simulink model "three_phase_diode_rectifier_with_input_filter"  (R2016a)
settings: Solver=VariableStepAuto  StartTime=0.0  StopTime=0.5  RelTol=1e-3
libraries: powerlib x54
settings Model: Creator=Gorkem  LastModifiedBy=Gorkem

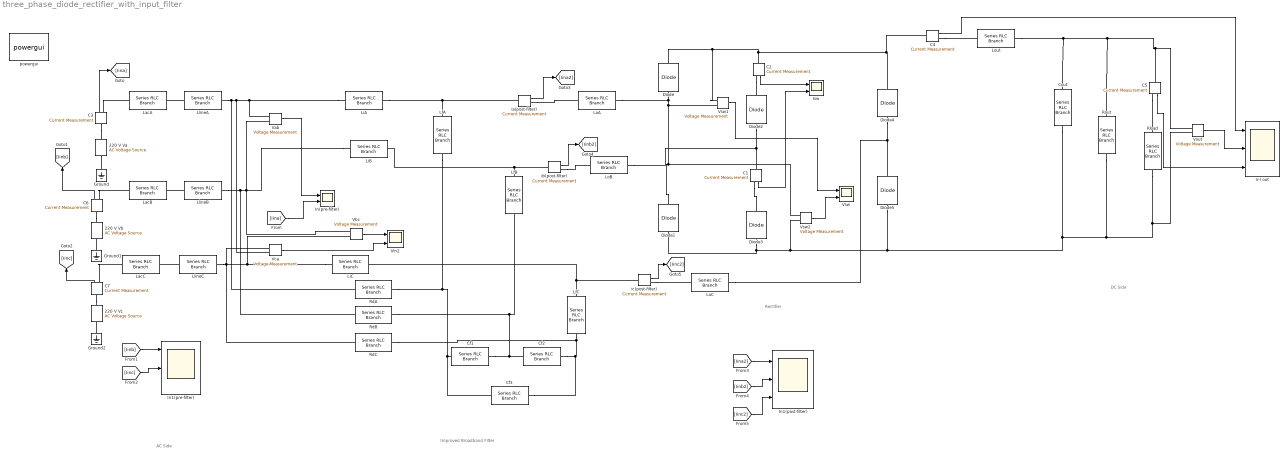
== system three_phase_diode_rectifier_with_input_filter ==
  note: Improved Broadband Filter
  note: DC Side
  note: Rectifier
  note: AC Side
  220 V Va : powerlib/Electrical Sources/AC Voltage Source  Amplitude=311  Phase=0  Frequency=50  SampleTime=0  Measurements=Voltage  BusType=swing  Pref=10e3  Qref=0  Qmin=-inf  Qmax=+inf
  220 V Vb : powerlib/Electrical Sources/AC Voltage Source  Amplitude=311  Phase=120  Frequency=50  SampleTime=0  Measurements=Voltage  BusType=swing  Pref=10e3  Qref=0  Qmin=-inf  Qmax=+inf
  220 V Vc : powerlib/Electrical Sources/AC Voltage Source  Amplitude=311  Phase=240  Frequency=50  SampleTime=0  Measurements=Voltage  BusType=swing  Pref=10e3  Qref=0  Qmin=-inf  Qmax=+inf
  C{1..7} (7 alike) : powerlib/Measurements/Current Measurement  PhasorSimulation=off  OutputType=Complex  PSBequivalent=0
  Cf1 : powerlib/Elements/Series RLC Branch  LConnTagsString=__new0  RConnTagsString=__new0  BranchType=C  Resistance=0.1  Inductance=1.7e-3  SetiL0=off  InitialCurrent=0  Capacitance=60e-6  Setx0=off  InitialVoltage=0  Measurements=Branch voltage and current
  Cf2 : powerlib/Elements/Series RLC Branch  LConnTagsString=__new0  RConnTagsString=__new0  BranchType=C  Resistance=0.1  Inductance=1.7e-3  SetiL0=off  InitialCurrent=0  Capacitance=60e-6  Setx0=off  InitialVoltage=0  Measurements=Branch voltage and current
  Cf3 : powerlib/Elements/Series RLC Branch  LConnTagsString=__new0  RConnTagsString=__new0  BranchType=C  Resistance=0.1  Inductance=1.7e-3  SetiL0=off  InitialCurrent=0  Capacitance=60e-6  Setx0=off  InitialVoltage=0  Measurements=Branch voltage and current
  Cout : powerlib/Elements/Series RLC Branch  LConnTagsString=__new0  RConnTagsString=__new0  BranchType=RC  Resistance=0.3  Inductance=1.6e-3  SetiL0=off  InitialCurrent=0  Capacitance=6e-3  Setx0=off  InitialVoltage=0  Measurements=Branch voltage and current
  Diode{,1..5} (6 alike) : powerlib/Power Electronics/Diode  Ron=0.01  Lon=0  Vf=0.7  IC=0  UseSnubber=off  Rs=5  Cs=0.1e-3  Measurements=off
  Ground : powerlib/Elements/Ground  LConnTagsString=a
  Ground1 : powerlib/Elements/Ground  LConnTagsString=a
  Ground2 : powerlib/Elements/Ground  LConnTagsString=a
  In(pre-filter) : Scope  NumInputPorts=2
  In1(post-filter) : Scope  NumInputPorts=3
  In1(pre-filter) : Scope  NumInputPorts=3
  Isw : Scope  NumInputPorts=2
  LacA : powerlib/Elements/Series RLC Branch  LConnTagsString=__new0  RConnTagsString=__new0  BranchType=RL  Resistance=0.1  Inductance=10e-3  SetiL0=off  InitialCurrent=0  Capacitance=1e-6  Setx0=off  InitialVoltage=0  Measurements=Branch voltage and current
  LacB : powerlib/Elements/Series RLC Branch  LConnTagsString=__new0  RConnTagsString=__new0  BranchType=RL  Resistance=0.1  Inductance=10e-3  SetiL0=off  InitialCurrent=0  Capacitance=1e-6  Setx0=off  InitialVoltage=0  Measurements=Branch voltage and current
  LacC : powerlib/Elements/Series RLC Branch  LConnTagsString=__new0  RConnTagsString=__new0  BranchType=RL  Resistance=0.1  Inductance=10e-3  SetiL0=off  InitialCurrent=0  Capacitance=1e-6  Setx0=off  InitialVoltage=0  Measurements=Branch voltage and current
  LfA : powerlib/Elements/Series RLC Branch  LConnTagsString=__new0  RConnTagsString=__new0  BranchType=L  Resistance=0.1  Inductance=1.7e-3  SetiL0=off  InitialCurrent=0  Capacitance=1e-6  Setx0=off  InitialVoltage=0  Measurements=Branch voltage and current
  LfB : powerlib/Elements/Series RLC Branch  LConnTagsString=__new0  RConnTagsString=__new0  BranchType=L  Resistance=0.1  Inductance=1.7e-3  SetiL0=off  InitialCurrent=0  Capacitance=1e-6  Setx0=off  InitialVoltage=0  Measurements=Branch voltage and current
  LfC : powerlib/Elements/Series RLC Branch  LConnTagsString=__new0  RConnTagsString=__new0  BranchType=L  Resistance=0.1  Inductance=1.7e-3  SetiL0=off  InitialCurrent=0  Capacitance=1e-6  Setx0=off  InitialVoltage=0  Measurements=Branch voltage and current
  LiA : powerlib/Elements/Series RLC Branch  LConnTagsString=__new0  RConnTagsString=__new0  BranchType=L  Resistance=0.1  Inductance=3.8e-3  SetiL0=off  InitialCurrent=0  Capacitance=1e-6  Setx0=off  InitialVoltage=0  Measurements=Branch voltage and current
  LiB : powerlib/Elements/Series RLC Branch  LConnTagsString=__new0  RConnTagsString=__new0  BranchType=L  Resistance=0.1  Inductance=3.8e-3  SetiL0=off  InitialCurrent=0  Capacitance=1e-6  Setx0=off  InitialVoltage=0  Measurements=Branch voltage and current
  LiC : powerlib/Elements/Series RLC Branch  LConnTagsString=__new0  RConnTagsString=__new0  BranchType=L  Resistance=0.1  Inductance=3.8e-3  SetiL0=off  InitialCurrent=0  Capacitance=1e-6  Setx0=off  InitialVoltage=0  Measurements=Branch voltage and current
  LlineA : powerlib/Elements/Series RLC Branch  LConnTagsString=__new0  RConnTagsString=__new0  BranchType=RL  Resistance=0.015  Inductance=5e-6  SetiL0=off  InitialCurrent=0  Capacitance=1e-6  Setx0=off  InitialVoltage=0  Measurements=Branch voltage and current
  LlineB : powerlib/Elements/Series RLC Branch  LConnTagsString=__new0  RConnTagsString=__new0  BranchType=RL  Resistance=0.015  Inductance=5e-6  SetiL0=off  InitialCurrent=0  Capacitance=1e-6  Setx0=off  InitialVoltage=0  Measurements=Branch voltage and current
  LlineC : powerlib/Elements/Series RLC Branch  LConnTagsString=__new0  RConnTagsString=__new0  BranchType=RL  Resistance=0.015  Inductance=5e-6  SetiL0=off  InitialCurrent=0  Capacitance=1e-6  Setx0=off  InitialVoltage=0  Measurements=Branch voltage and current
  LoA : powerlib/Elements/Series RLC Branch  LConnTagsString=__new0  RConnTagsString=__new0  BranchType=L  Resistance=0.1  Inductance=1.1e-3  SetiL0=off  InitialCurrent=0  Capacitance=1e-6  Setx0=off  InitialVoltage=0  Measurements=Branch voltage and current
  LoB : powerlib/Elements/Series RLC Branch  LConnTagsString=__new0  RConnTagsString=__new0  BranchType=L  Resistance=0.1  Inductance=1.1e-3  SetiL0=off  InitialCurrent=0  Capacitance=1e-6  Setx0=off  InitialVoltage=0  Measurements=Branch voltage and current
  LoC : powerlib/Elements/Series RLC Branch  LConnTagsString=__new0  RConnTagsString=__new0  BranchType=L  Resistance=0.1  Inductance=1.1e-3  SetiL0=off  InitialCurrent=0  Capacitance=1e-6  Setx0=off  InitialVoltage=0  Measurements=Branch voltage and current
  "Lout " : powerlib/Elements/Series RLC Branch  LConnTagsString=__new0  RConnTagsString=__new0  BranchType=RL  Resistance=0.2e-3  Inductance=20e-3  SetiL0=off  InitialCurrent=0  Capacitance=1e-6  Setx0=off  InitialVoltage=0  Measurements=Branch voltage and current
  RdA : powerlib/Elements/Series RLC Branch  LConnTagsString=__new0  RConnTagsString=__new0  BranchType=R  Resistance=10  Inductance=10e-3  SetiL0=off  InitialCurrent=0  Capacitance=1e-6  Setx0=off  InitialVoltage=0  Measurements=Branch voltage and current
  RdB : powerlib/Elements/Series RLC Branch  LConnTagsString=__new0  RConnTagsString=__new0  BranchType=R  Resistance=10  Inductance=10e-3  SetiL0=off  InitialCurrent=0  Capacitance=1e-6  Setx0=off  InitialVoltage=0  Measurements=Branch voltage and current
  RdC : powerlib/Elements/Series RLC Branch  LConnTagsString=__new0  RConnTagsString=__new0  BranchType=R  Resistance=10  Inductance=10e-3  SetiL0=off  InitialCurrent=0  Capacitance=1e-6  Setx0=off  InitialVoltage=0  Measurements=Branch voltage and current
  Rload : powerlib/Elements/Series RLC Branch  LConnTagsString=__new0  RConnTagsString=__new0  BranchType=R  Resistance=150  Inductance=1.6e-3  SetiL0=off  InitialCurrent=0  Capacitance=1e-6  Setx0=off  InitialVoltage=0  Measurements=Branch voltage and current
  Rout : powerlib/Elements/Series RLC Branch  LConnTagsString=__new0  RConnTagsString=__new0  BranchType=R  Resistance=10  Inductance=1.6e-3  SetiL0=off  InitialCurrent=0  Capacitance=1e-6  Setx0=off  InitialVoltage=0  Measurements=Branch voltage and current
  V-I out : Scope  NumInputPorts=3
  Vab : powerlib/Measurements/Voltage Measurement  PhasorSimulation=off  OutputType=Complex  PSBequivalent=0
  Vbc : powerlib/Measurements/Voltage Measurement  PhasorSimulation=off  OutputType=Complex  PSBequivalent=0
  Vca : powerlib/Measurements/Voltage Measurement  PhasorSimulation=off  OutputType=Complex  PSBequivalent=0
  Vin2 : Scope  NumInputPorts=2
  Vout : powerlib/Measurements/Voltage Measurement  PhasorSimulation=off  OutputType=Complex  PSBequivalent=0
  Vsw : Scope  NumInputPorts=2
  Vsw1 : powerlib/Measurements/Voltage Measurement  PhasorSimulation=off  OutputType=Complex  PSBequivalent=0
  Vsw2 : powerlib/Measurements/Voltage Measurement  PhasorSimulation=off  OutputType=Complex  PSBequivalent=0
  ia(post-filter) : powerlib/Measurements/Current Measurement  PhasorSimulation=off  OutputType=Complex  PSBequivalent=0
  ib(post-filter) : powerlib/Measurements/Current Measurement  PhasorSimulation=off  OutputType=Complex  PSBequivalent=0
  ic(post-filter) : powerlib/Measurements/Current Measurement  PhasorSimulation=off  OutputType=Complex  PSBequivalent=0
  powergui : powerlib/powergui  Priority=1  SimulationMode=Continuous  SolverType=Tustin/Backward Euler (TBE)  SampleTime=50e-6  frequency=60  SPID=off  DisableSnubberDevices=on  DisableRonSwitches=off  DisableVfSwitches=off  SwTol=0  DisplayEquations=off  Interpol=off  ExternalGateDelay=off  methode=off  Ts=10  FunctionMessages=on  echomessages=on  HookPort=off  EnableUseOfTLC=off  x0status=blocks  frequencyindice=0  Pbase=250  ErrMax=1e-4  Iterations=50  UnitsV=V  UnitsW=W  buscounter=0  RestoreLinks=warning  ResistiveCurrentMeasurement=off  Frange=[0:2:500]  Ylog=off  Xlog=on  ShowGrid=off  save=off  variable=ZData  structure=0  ZoomFFT=off  StartTime=0.0  cycles=1  DisplayStyle=1  fundamental=60  FreqAxis=off  MaxFrequency=1000  frequencyindicesteady=1  RmsSteady=1  display=off
  wires:
  Vab/1 -> In(pre-filter)/1
  C2/1 -> Isw/1
  C1/1 -> Isw/2
  C3/1 -> [Iina]
  [Iina] -> In(pre-filter)/2
  Vout/1 -> V-I out/2
  C4/1 -> V-I out/1
  Vsw1/1 -> Vsw/1
  Vsw2/1 -> Vsw/2
  C5/1 -> V-I out/3
  [Iinb] -> In1(pre-filter)/1
  [Iinc] -> In1(pre-filter)/2
  C6/1 -> [Iinb]
  C7/1 -> [Iinc]
  Vbc/1 -> Vin2/1
  Vca/1 -> Vin2/2
  ia(post-filter)/1 -> [Iina2]
  ib(post-filter)/1 -> [Iinb2]
  ic(post-filter)/1 -> [Iinc2]
  [Iina2] -> In1(post-filter)/1
  [Iinb2] -> In1(post-filter)/2
  [Iinc2] -> In1(post-filter)/3
  connections:
  LlineA/LConn1 -- LacA/RConn1
  Diode4/RConn1 -- C4/LConn1 -- Diode/RConn1 -- Vsw1/LConn1 -- C2/LConn1
  Diode3/LConn1 -- Rout/RConn1 -- Vout/LConn2 -- Rload/RConn1 -- Cout/RConn1 -- Diode5/LConn1 -- Vsw2/LConn2 -- Diode1/LConn1
  LiA/LConn1 -- LlineA/RConn1 -- RdA/LConn1 -- Vca/LConn2 -- Vab/LConn1
  C2/RConn1 -- Diode2/RConn1
  C3/LConn1 -- 220 V Va/RConn1
  C3/RConn1 -- LacA/LConn1
  "Lout "/RConn1 -- Cout/LConn1 -- Rout/LConn1 -- C5/LConn1 -- Vout/LConn1
  LiB/LConn1 -- RdB/LConn1 -- LlineB/RConn1 -- Vbc/LConn1 -- Vab/LConn2
  C1/RConn1 -- Diode3/RConn1
  C5/RConn1 -- Rload/LConn1
  LiC/LConn1 -- RdC/LConn1 -- Vca/LConn1 -- LlineC/RConn1 -- Vbc/LConn2
  Ground/LConn1 -- 220 V Va/LConn1
  Ground1/LConn1 -- 220 V Vb/LConn1
  Ground2/LConn1 -- 220 V Vc/LConn1
  C6/LConn1 -- 220 V Vb/RConn1
  LlineB/LConn1 -- LacB/RConn1
  C7/LConn1 -- 220 V Vc/RConn1
  LlineC/LConn1 -- LacC/RConn1
  C4/RConn1 -- "Lout "/LConn1
  Vsw1/LConn2 -- LoA/RConn1 -- Diode/LConn1 -- Vsw2/LConn1 -- Diode1/RConn1
  Diode2/LConn1 -- LoB/RConn1 -- C1/LConn1
  Diode4/LConn1 -- LoC/RConn1 -- Diode5/RConn1
  LfA/RConn1 -- Cf3/RConn1 -- Cf1/RConn1 -- RdA/RConn1
  Cf2/RConn1 -- Cf1/LConn1 -- RdB/RConn1 -- LfB/RConn1
  Cf2/LConn1 -- Cf3/LConn1 -- RdC/RConn1 -- LfC/RConn1
  LiA/RConn1 -- ia(post-filter)/LConn1 -- LfA/LConn1
  LfB/LConn1 -- LiB/RConn1 -- ib(post-filter)/LConn1
  LfC/LConn1 -- ic(post-filter)/LConn1 -- LiC/RConn1
  LacB/LConn1 -- C6/RConn1
  LacC/LConn1 -- C7/RConn1
  ia(post-filter)/RConn1 -- LoA/LConn1
  ib(post-filter)/RConn1 -- LoB/LConn1
  ic(post-filter)/RConn1 -- LoC/LConn1
